simulink model "OL_fullnonlin_prevval_ucorr"  (R2024b)
settings: Solver=VariableStepAuto  StartTime=0.0  StopTime=10.0  RelTol=1e-3
undefined symbols (not defined in the file): pars
settings Model: Creator=kkajak  LastModifiedBy=feder
settings SolverCC: AlgebraicLoopSolver=TrustRegion
settings DataIOCC: ExternalInput=OL_fullnonlin_statederiv_test.getElement(1)  LoadExternalInput=on  ReturnWorkspaceOutputs=off
settings DebuggingCC: UnconnectedInputMsg=warning  UnconnectedOutputMsg=warning  UnconnectedLineMsg=warning  ArithmeticOperatorsInVariantConditions=warning
settings ModelReferenceCC: EnableRefExpFcnMdlSchedulingChecks=on
settings SFSimCC: SimUseLocalCustomCode=off  CustomCodeUndefinedFunction=UseInterfaceOnly
settings RTWCC: RTWUseLocalCustomCode=off  GPUComputeCapability=3.5
settings CodeAppCC: StateflowObjectComments=on

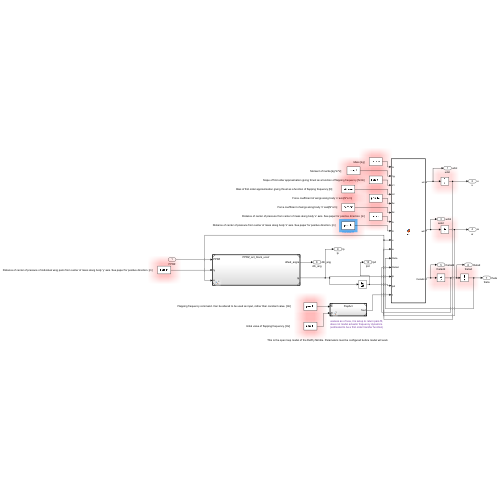
[thumbnail: Simulink's stored preview of the top-level diagram]
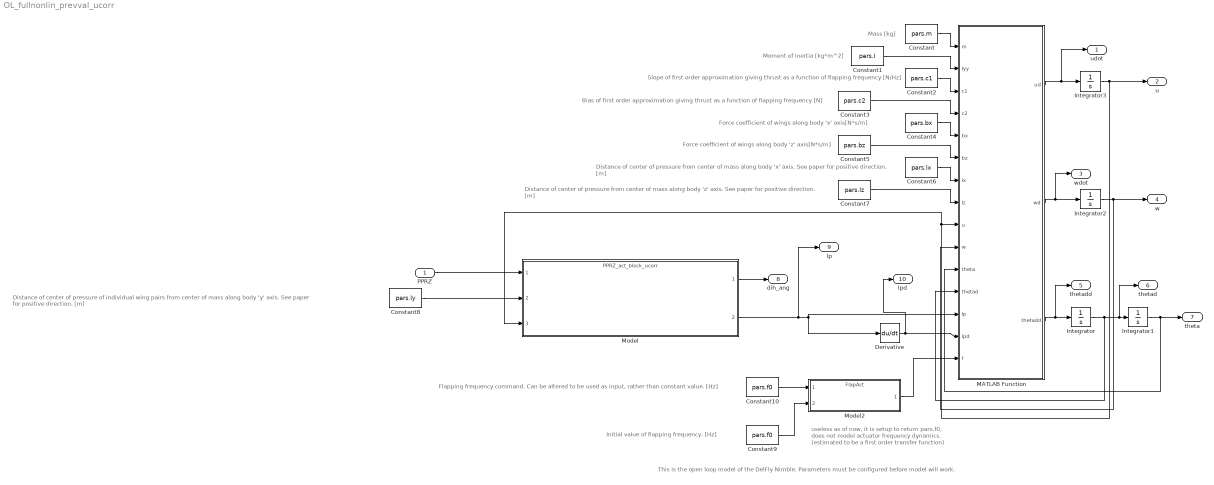
== system OL_fullnonlin_prevval_ucorr ==
  note: Initial value of flapping frequency. [Hz]
  note: Flapping frequency command. Can be altered to be used as input, rather than constant value. [Hz]
  note: Distance of center of pressure from center of mass along body 'x' axis. See paper for positive direction. [m]
  note: Force coefficient of wings along body 'x' axis[N*s/m]
  note: Slope of first order approximation giving thrust as a function of flapping frequency [N/Hz]
  note: Moment of inertia [kg*m^2]
  note: Mass [kg]
  note: This is the open loop model of the DelFly Nimble. Parameters must be configured before model will work.
  note: Bias of first order approximation giving thrust as a function of flapping frequency [N]
  note: Force coefficient of wings along body 'z' axis[N*s/m]
  note: Distance of center of pressure from center of mass along body 'z' axis. See paper for positive direction. [m]
  note: Distance of center of pressure of individual wing pairs from center of mass along body 'y' axis. See paper for positive direction. [m]
  note: useless as of now, it is setup to return pars.f0,
      | does not model actuator frequency dynamics.
      | (estimated to be a first order transfer function)
  PPRZ : Inport
  Constant : Constant  Value=pars.m
  Constant1 : Constant  Value=pars.I
  Constant10 : Constant  Value=pars.f0
  Constant2 : Constant  Value=pars.c1
  Constant3 : Constant  Value=pars.c2
  Constant4 : Constant  Value=pars.bx
  Constant5 : Constant  Value=pars.bz
  Constant6 : Constant  Value=pars.lx
  Constant7 : Constant  Value=pars.lz
  Constant8 : Constant  Value=pars.ly
  Constant9 : Constant  Value=pars.f0
  Derivative : Derivative
  Integrator : Integrator  InitialCondition=pars.thetad0
  Integrator1 : Integrator  InitialCondition=pars.theta0
  Integrator2 : Integrator  InitialCondition=pars.w0
  Integrator3 : Integrator  InitialCondition=pars.u0
  MATLAB Function : MATLAB Function  TreatAsAtomicUnit=on
  Model : ModelReference  ModelNameDialog=PPRZ_act_block_ucorr  SimulationMode=Normal  ModelReferenceVersion=1.8
  Model2 : ModelReference  ModelNameDialog=FlapAct  SimulationMode=Normal  ModelReferenceVersion=1.2
  udot : Outport  SignalName=udot
  u : Outport  Port=2  SignalName=u
  wdot : Outport  Port=3  SignalName=wdot
  w : Outport  Port=4  SignalName=w
  thetadd : Outport  Port=5  SignalName=thetadd
  thetad : Outport  Port=6  SignalName=thetad
  theta : Outport  Port=7  SignalName=theta
  dih_ang : Outport  Port=8  SignalName=dih_ang
  lp : Outport  Port=9  SignalName=lp
  lpd : Outport  Port=10  SignalName=lpd
  wires:
  Constant/1 -> MATLAB Function/1(m)
  Constant1/1 -> MATLAB Function/2(Iyy)
  Constant2/1 -> MATLAB Function/3(c1)
  Constant3/1 -> MATLAB Function/4(c2)
  Constant4/1 -> MATLAB Function/5(bx)
  Constant5/1 -> MATLAB Function/6(bz)
  Constant6/1 -> MATLAB Function/7(lx)
  Constant7/1 -> MATLAB Function/8(lz)
  MATLAB Function/3(thetadd) -> thetadd/1, Integrator/1
  Integrator1/1 -> theta/1, MATLAB Function/11(theta)
  Integrator/1 -> MATLAB Function/12(thetad), thetad/1, Integrator1/1
  MATLAB Function/2(wd) -> wdot/1, Integrator2/1
  Integrator2/1 -> w/1, MATLAB Function/10(w)
  MATLAB Function/1(ud) -> udot/1, Integrator3/1
  Integrator3/1 -> u/1, Model/3, MATLAB Function/9(u)
  Derivative/1 -> lpd/1, MATLAB Function/14(lpd)
  Model2/1 -> MATLAB Function/15(f)
  Constant9/1 -> Model2/2
  Constant10/1 -> Model2/1
  Model/1 -> dih_ang/1
  PPRZ/1 -> Model/1
  Constant8/1 -> Model/2
  Model/2 -> lp/1, MATLAB Function/13(lp), Derivative/1

== matlab function OL_fullnonlin_prevval_ucorr/MATLAB Function ==
  data: m input; Iyy input; c1 input; c2 input; bx input; bz input; lx input; lz input; u input; ud output; w input; theta input; thetad input; lp input; lpd input; wd output; thetadd output; f input
function [ud,wd,thetadd] = fcn(m,Iyy, c1, c2, bx, bz, lx, lz, u, w, theta, thetad, lp, lpd, f)





  
g = 9.80665;
ud = -sin(theta)*g - 2*bx/m*u + lz*2*bx*thetad/m + 2*bx*lpd/m - thetad*w;
% % % ud = -sin(theta)*g - 2*bx/m*u + lz*2*bx*thetad/m + 2*bx*lpd/m;
% % 
wd = cos(theta)*g - 2*(c1*f + c2)/m - 2*bz*w/m - 2*bz*(lp+lx)*thetad/m + thetad*u;   
% % % wd = cos(theta)*g - 2*(c1*f + c2)/m - 2*bz*w/m - 2*bz*(lp+lx)*thetad/m;  
% 
thetadd = (2*bx*lz*u - 2*bx*lz^2*(thetad) - 2*bx*lz*(lpd)...
 - 2*c1*f.*(lp+lx) - 2*c2*(lp+lx) - 2*bz*w.*(lp+lx) - 2*bz*(lp+lx).^2.*(thetad))/Iyy;




% ud = -sin(theta)*g - 2*bx/m*u + lz*2*bx*thetad/m + 2*bx*f*lpd/m - thetad*w;
% ud = -sin(theta)*g - 2*bx/m*u + lz*2*bx*thetad/m + 2*bx*lpd/m;
% 
% wd = cos(theta)*g - 2*(c1*f + c2)/m - 2*bz*w/m - 2*bz*f*(lp+lx)*thetad/m + thetad*u;   
%wd = cos(theta)*g - 2*(c1*f + c2)/m - 2*bz*w/m - 2*bz*(lp)*thetad/m;  
% 
% thetadd = (2*bx*lz*u - 2*bx*lz^2*(thetad) - 2*bx*lz*(lpd)...
% - 2*c1*f.*(lp+lx) - 2*c2*(lp) - 2*bz*w.*(lp) - 2*bz*(lp).^2.*(thetad))/Iyy;
end
% % X = -2*bx*u + lz*2*bx*thetad + 2*bx*lpd;
% % X = -2*bx*u + lz*2*bx*thetad;
% X = -2*bx*u;
% Z = - 2*(c1*f + c2) - 2*bz*w - 2*bz*(lp+lx)*thetad;
% 
% l = [-lx-lp; 0; -lz];
% M = -cross([X;0;Z],l);
% My = M(2);
% 
% ud = -g*sin(theta) + X/m - thetad*w;
% wd = g*cos(theta) + Z/m + thetad*u;
% % ud = -g*sin(theta) + X/m;
% % wd = g*cos(theta) + Z/m;
% thetadd = My/Iyy;
